simulink model "popul"  (Simulink 8.7)
settings: Solver=VariableStepAuto  StartTime=0.0  StopTime=10  RelTol=1e-3
settings Model: Creator=Dinis  LastModifiedBy=Dinis  SimulationMode=accelerator
settings DataIOCC: LimitDataPoints=off  SaveFormat=Dataset
settings DebuggingCC: UnderspecifiedInitializationDetection=Simplified  MergeDetectMultiDrivingBlocksExec=error
settings HardwareCC: ProdBitPerPointer=64  ProdLargestAtomicFloat=Float  ProdIntDivRoundTo=Zero  ProdEndianess=LittleEndian  ProdWordSize=64  ProdHWDeviceType=Intel->x86-64 (Windows64)
settings ModelReferenceCC: PropagateSignalLabelsOutOfModel=on
settings ConfigComp: CovModelRefEnable=off

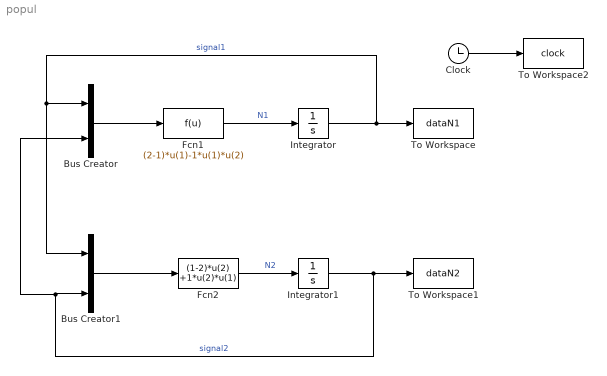
== system popul ==
  Bus Creator : BusCreator  Inputs=2
  Bus Creator1 : BusCreator  Inputs=2
  Clock : Clock
  Fcn1 : Fcn  Expr=(2-1)*u(1)-1*u(1)*u(2)
  Fcn2 : Fcn  Expr=(1-2)*u(2) +1*u(2)*u(1)
  Integrator : Integrator  InitialCondition=2
  Integrator1 : Integrator  InitialCondition=2
  To Workspace : ToWorkspace  VariableName=dataN1  SaveFormat=Timeseries  SampleTime=-1
  To Workspace1 : ToWorkspace  VariableName=dataN2  SaveFormat=Timeseries  SampleTime=-1
  To Workspace2 : ToWorkspace  VariableName=clock  SaveFormat=Timeseries  SampleTime=-1
  wires:
  Bus Creator1/1 -> Fcn2/1
  Fcn2/1 -> Integrator1/1  "N2"
  Fcn1/1 -> Integrator/1  "N1"
  Bus Creator/1 -> Fcn1/1
  Integrator/1 -> Bus Creator1/1, Bus Creator/1, To Workspace/1  "signal1"
  Integrator1/1 -> Bus Creator/2, Bus Creator1/2, To Workspace1/1  "signal2"
  Clock/1 -> To Workspace2/1
